simulink model "BraytonCycle"  (R2015a)
settings: Solver=ode45  StartTime=0.0  StopTime=10.0  RelTol=1e-3
libraries: Lib_Thermo_PT2S_TMATS x2, Lib_Thermo_SP2T_TMATS x2, Lib_Thermo_Enth2Temp_TMATS x1, Lib_Thermo_Temp2Enth_TMATS x1
settings Model: Creator=jwchapm2  LastModifiedBy=jwchapm2

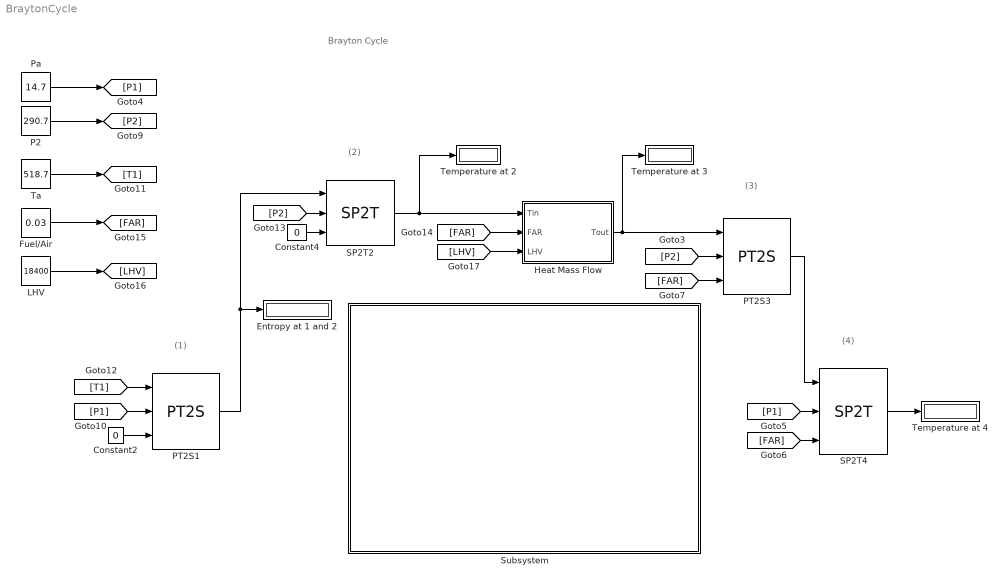
== system BraytonCycle ==
  note: Brayton Cycle
  note: (1)
  note: (2)
  note: (3)
  note: (4)
  Constant2 : Constant  Value=0
  Constant4 : Constant  Value=0
  Entropy at 1 and 2 : Display
  Fuel/Air : Constant  Value=0.03
  Heat Mass Flow : Subsystem
  LHV : Constant  Value=18400
  P2 : Constant  Value=290.7
  PT2S1 : Lib_Thermo_PT2S_TMATS/PT2S
  PT2S3 : Lib_Thermo_PT2S_TMATS/PT2S
  Pa : Constant  Value=14.7
  SP2T2 : Lib_Thermo_SP2T_TMATS/SP2T
  SP2T4 : Lib_Thermo_SP2T_TMATS/SP2T
  Subsystem : Subsystem
      mask Display: image(imread(which('TMATS_brayton.jpg')))
  Ta : Constant  Value=518.7
  Temperature at 2 : Display
  Temperature at 3 : Display
  Temperature at 4 : Display
  wires:
  PT2S1/1 -> SP2T2/1, Entropy at 1 and 2/1
  [T1] -> PT2S1/1
  Constant2/1 -> PT2S1/3
  Constant4/1 -> SP2T2/3
  SP2T2/1 -> Temperature at 2/1, Heat Mass Flow/1(Tin)
  [P2] -> PT2S3/2
  PT2S3/1 -> SP2T4/1
  [P1] -> SP2T4/2
  [FAR] -> SP2T4/3
  [FAR] -> PT2S3/3
  SP2T4/1 -> Temperature at 4/1
  [P1] -> PT2S1/2
  Pa/1 -> [P1]
  P2/1 -> [P2]
  Ta/1 -> [T1]
  [P2] -> SP2T2/2
  Fuel/Air/1 -> [FAR]
  LHV/1 -> [LHV]
  Heat Mass Flow/1(Tout) -> PT2S3/1, Temperature at 3/1
  [FAR] -> Heat Mass Flow/2(FAR)
  [LHV] -> Heat Mass Flow/3(LHV)

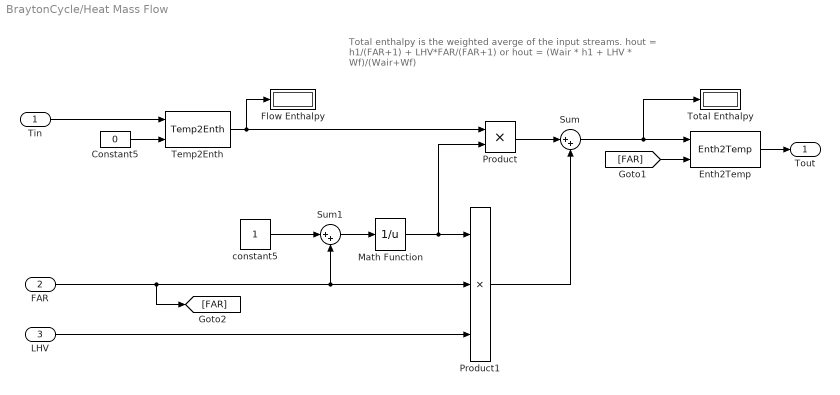
== system BraytonCycle/Heat Mass Flow ==
  note: Total enthalpy is the weighted averge of the input streams.
      |
      | hout = h1/(FAR+1) + LHV*FAR/(FAR+1)
      | 				or
      | hout = (Wair * h1 + LHV * Wf)/(Wair+Wf)
  Tin : Inport
  FAR : Inport  Port=2
  LHV : Inport  Port=3
  Constant5 : Constant  Value=0
  Enth2Temp : Lib_Thermo_Enth2Temp_TMATS/Enth2Temp
  Flow Enthalpy : Display
  Math Function : Math  Operator=reciprocal  SaturateOnIntegerOverflow=on
  Product : Product
  Product1 : Product  Inputs=3
  Sum : Sum  Inputs=|++
  Sum1 : Sum  Inputs=|++
  Temp2Enth : Lib_Thermo_Temp2Enth_TMATS/Temp2Enth
  Total Enthalpy : Display
  constant5 : Constant
  Tout : Outport
  wires:
  Sum1/1 -> Math Function/1
  Product/1 -> Sum/1
  Math Function/1 -> Product1/1, Product/2
  Sum/1 -> Total Enthalpy/1, Enth2Temp/1
  LHV/1 -> Product1/3
  constant5/1 -> Sum1/1
  Enth2Temp/1 -> Tout/1
  [FAR] -> Enth2Temp/2
  Constant5/1 -> Temp2Enth/2
  Temp2Enth/1 -> Flow Enthalpy/1, Product/1
  Tin/1 -> Temp2Enth/1
  Product1/1 -> Sum/2
  FAR/1 -> [FAR], Sum1/2, Product1/2

== system BraytonCycle/Subsystem ==
